simulink model "W01_S3"  (R2024b)
settings: Solver=ode4  StartTime=0  StopTime=T_final  FixedStep=h  RelTol=1e-3
undefined symbols (not defined in the file or in its folder): beta_c, mp, n0, rp, V_c, x0
settings Model: Creator=admin  LastModifiedBy=admin
settings DataIOCC: ReturnWorkspaceOutputs=off

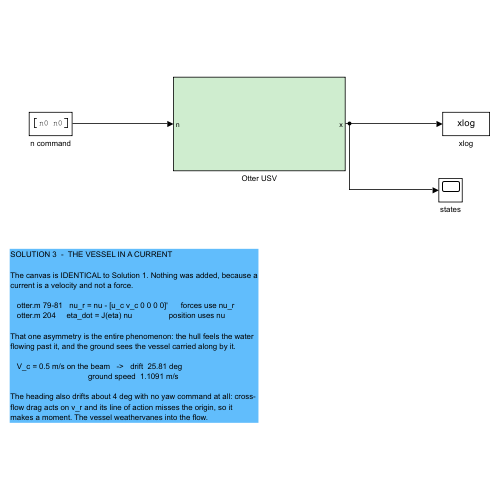
[thumbnail: Simulink's stored preview of the top-level diagram]
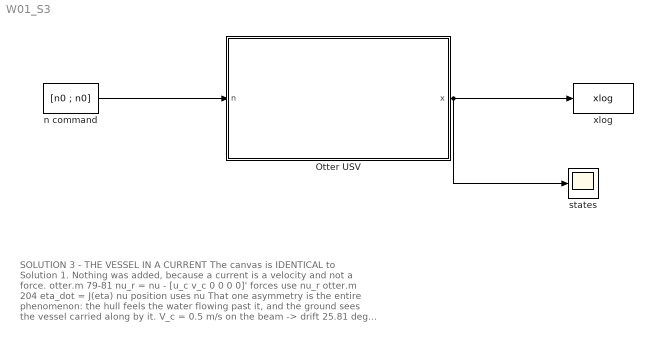
== system W01_S3 ==
  note: SOLUTION 3  -  THE VESSEL IN A CURRENT
      |
      | The canvas is IDENTICAL to Solution 1. Nothing was added, because a
      | current is a velocity and not a force.
      |
      |    otter.m 79-81   nu_r = nu - [u_c v_c 0 0 0 0]'      forces use nu_r
      |    otter.m 204     eta_dot = J(eta) nu                 position uses nu
      |
      | That one asymmetry is the entire phenomenon: the hull feels the water
      | flowing past it, and the ground sees the vessel carried along by it.
      |
      |    V_c = 0.5 m/s on the beam   ->   drift  25.81 deg
      |                                     ground speed  1.1091 m/s
      |
      | The heading also drifts about 4 deg with no yaw command at all: cross-
      | flow drag acts on v_r and its line of action misses the origin, so it
      | makes a moment. The vessel weathervanes into the flow.
  Otter USV : Subsystem
  n command : Constant  Value=[n0 ; n0]
  states : Scope
  xlog : ToWorkspace  VariableName=xlog  SaveFormat=Structure With Time  SampleTime=-1
  wires:
  n command/1 -> Otter USV/1(n)
  Otter USV/1(x) -> xlog/1, states/1

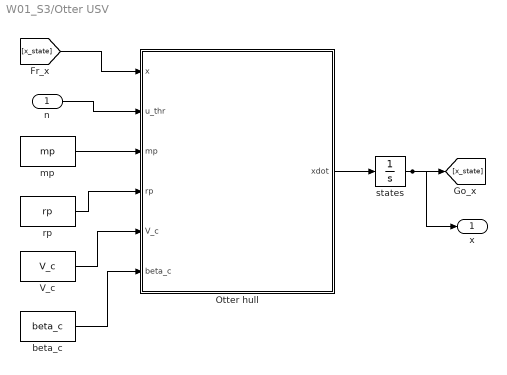
== system W01_S3/Otter USV ==
  n : Inport
  Otter hull : MATLAB Function  TreatAsAtomicUnit=on
  V_c : Constant  Value=V_c
  beta_c : Constant  Value=beta_c
  mp : Constant  Value=mp
  rp : Constant  Value=rp
  states : Integrator  InitialCondition=x0
  x : Outport
  wires:
  [x_state] -> Otter hull/1(x)
  n/1 -> Otter hull/2(u_thr)
  rp/1 -> Otter hull/4(rp)
  mp/1 -> Otter hull/3(mp)
  V_c/1 -> Otter hull/5(V_c)
  states/1 -> [x_state], x/1
  beta_c/1 -> Otter hull/6(beta_c)
  Otter hull/1(xdot) -> states/1

== matlab function W01_S3/Otter USV/Otter hull ==
  data: x input; xdot output double size=[12 1]; u_thr input; mp input; rp input; V_c input; beta_c input
function xdot = otter_hull(x, u_thr, mp, rp, V_c, beta_c)
% Fossen's otter.m, called unchanged from Tools/MSS/VESSELS.
%
%   x       12 states, fed back from the integrator
%   u_thr   propeller shaft speeds [rad/s]
%
% otter.m is not written for code generation, so the call is extrinsic and
% xdot has to be pre-sized for Simulink to know the output width.
coder.extrinsic('otter');

xdot = zeros(12,1);
xdot = otter(x, u_thr, mp, rp, V_c, beta_c);
end
